simulink model "lmsadeq"  (Simulink 6.0)
settings: Solver=FixedStepDiscrete  SolverMode=SingleTasking  StartTime=0.0  StopTime=1000  RelTol=1e-3  AbsTol=1e-6
libraries: simulink x2, dspsnks4 x2, dspsigops x1, dsparch4 x1, dspsigattribs x1, dspadpt3 x1
settings Model: RequirementInfo=9  CovMetricSettings=d  Creator=don  LastModifiedBy=sconahan  ExtModeTrigMode=oneshot  ExtModeArmWhenConnect=off
settings DataIOCC: LimitDataPoints=off  SaveOutput=off  SaveTime=off  SignalLoggingName=sigsOut
settings OptimizationCC: BlockReduction=off  BooleanDataType=off  MultiInstanced=off  RollThreshold=2
settings FormatCC: IgnoreBidirectionalLines=off
settings DebuggingCC: IntegerOverflowMsg=none
settings HardwareCC: TargetUnknown=on
settings CodeAppCC: FileBanners=off  CustomSymbols=off
settings GRTTargetCC: TargetFcnLib=iso_c_tmw.mat  IsERTTarget=off

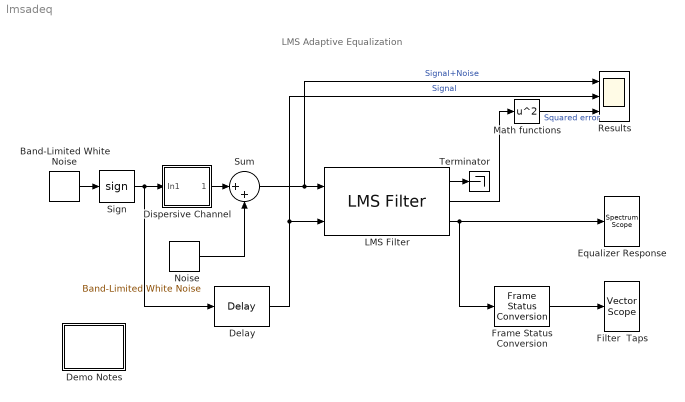
== system lmsadeq ==
  note: LMS Adaptive Equalization
  Band-Limited White Noise : simulink/Sources/Band-Limited White Noise  Cov=1e-5  Ts=1e-5  seed=12345
  Delay : dspsigops/Delay  dly_unit=Samples  delay=6  ic_detail=off  dif_ic_for_ch=off  dif_ic_for_dly=off  ic=0  reset_popup=None
  Demo Notes : Subsystem
      mask Display: disp('Notes')
  Dispersive Channel : Subsystem  mask(Simple Dispersive Channel){d=3.5}
      mask prompts: d "Dispersion:"
      mask help: Dispersive channel filter.
      mask init:
      | b=.5*(1+cos(2*pi./d.*[-1 0 1])); h=log(abs(freqz(b,1,64)));
      mask Help: Dispersive channel filter
      mask Display: plot(h)
  Equalizer Response : dspsnks4/Spectrum Scope  ScopeProperties=on  Domain=Frequency  HorizSpan=1  UseBuffer=off  BufferSize=128  Overlap=64  inpFftLenInherit=on  FFTlength=128  numAvg=2  DisplayProperties=off  AxisGrid=on  Memory=off  FrameNumber=off  AxisLegend=off  AxisZoom=off  OpenScopeAtSimStart=on  OpenScopeImmediately=off  FigPos=[29 124 450 360]  AxisProperties=off  XUnits=Hertz  XRange=[0...Fs/2]  InheritXIncr=on  XIncr=1  XLabel=Samples  YUnits=dB  YLabel=Magnitude, dB  LineProperties=off
      settings: YMin=-12  YMax=8
  Filter  Taps : dspsnks4/Vector Scope  ScopeProperties=on  Domain=User-defined  HorizSpan=1  DisplayProperties=off  AxisGrid=on  Memory=off  FrameNumber=off  AxisLegend=off  AxisZoom=off  OpenScopeAtSimStart=on  OpenScopeImmediately=off  FigPos=[491 123 450 360]  AxisProperties=off  XUnits=Hertz  XRange=[0...Fs/2]  InheritXIncr=off  XIncr=1  XLabel=Samples  YUnits=dB  YLabel=Equalizer Coefficients  LineProperties=off  LineMarkers=.
      settings: YMin=-1  YMax=2
  Frame Status Conversion : dspsigattribs/Frame Status Conversion  growRefPort=off  outframe=Frame-based
  LMS Filter : dspadpt3/LMS Filter  Algo=Normalized LMS  L=11  stepflag=Dialog  mu=0.5  leakage=1.0  addnparflag=off  ic=0  Adapt=off  resetflag=None  weights=on
  Math functions : Math  Operator=square  SaturateOnIntegerOverflow=on
  Noise : simulink/Sources/Band-Limited White Noise  Cov=.002e-5  Ts=1e-5  seed=[23341]
  Results : Scope  NumInputPorts=3
      settings: TimeRange=0.005  YMin=-2~0~0  YMax=2~2~1  DataFormat=Array
  Sign : Signum
  Sum : Sum  Inputs=|++  SaturateOnIntegerOverflow=on  InputSameDT=on
  Terminator : Terminator
  wires:
  LMS Filter/3 -> Frame Status Conversion/1, Equalizer Response/1
  Dispersive Channel/1(Out1) -> Sum/1
  Band-Limited White Noise/1 -> Sign/1
  Noise/1 -> Sum/2
  Sign/1 -> Dispersive Channel/1(In1), Delay/1
  LMS Filter/2 -> Math functions/1
  Math functions/1 -> Results/3  "Squared error"
  Delay/1 -> LMS Filter/2, Results/2  "Signal"
  Frame Status Conversion/1 -> Filter  Taps/1
  LMS Filter/1 -> Terminator/1
  Sum/1 -> LMS Filter/1, Results/1  "Signal+Noise"

== system lmsadeq/Demo Notes ==
  note: Adaptive Channel Equalization
      |
      | This demonstrates the ability of the LMS algorithm
      | to adaptively compute the estimate of an FIR
      | equalization filter.
      |
      | For more information on the LMS adaptive filter
      | or channel equalization, see
      | S. Haykin, "Adaptive Filter Theory",
      | 3rd Ed., Prentice Hall, 1996.

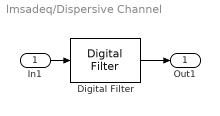
== system lmsadeq/Dispersive Channel ==
  In1 : Inport
  Digital Filter : dsparch4/Digital Filter  TypePopup=FIR (all zeros)  IIRFiltStruct=Direct form II transposed  AllPoleFiltStruct=Direct form  FIRFiltStruct=Direct form  CoeffSource=Specify via dialog  NumCoeffs=b  DenCoeffs=[1 0.1]  BiQuadCoeffs=[1 0.3 0.4 1 0.1 0.2]  LatticeCoeffs=[0.2 0.4]  denIgnore=on  FiltPerSampPopup=One filter per frame  IC=0  ICnum=0  ICden=0  roundingMode=Floor  overflowMode=off
  Out1 : Outport
  wires:
  Digital Filter/1 -> Out1/1
  In1/1 -> Digital Filter/1
